simulink subsystem "AeroPropRefFranc"  (R2024b)
settings: Solver=VariableStepAuto  StartTime=0.0  StopTime=10.0  RelTol=1e-3
undefined symbols (not defined in the file or in its folder): ess, Force_b, Fprop_r, geom, H_b, Hdot_b, Moment_b, mot, mot2, mot3, mot4, Mprop_r, propel, propel2, propel3, propel4, pxf_diagram_options, SimIn, SimPar, tc, tc2, tc3, tc4
libraries: simulink x8, slpidlib x4, starslibAxisTransformations x2, libAxisTransformations x2
(part 1 of 10)
settings Model: Creator=drhill  LastModifiedBy=adcl
settings SolverCC: AlgebraicLoopSolver=TrustRegion
settings OptimizationCC: ReuseModelBlockBuffer=off
settings DebuggingCC: UnconnectedInputMsg=warning  UnconnectedOutputMsg=warning  UnconnectedLineMsg=warning
settings ModelReferenceCC: EnableRefExpFcnMdlSchedulingChecks=on
settings RTWCC: GPUComputeCapability=3.5  DLArmComputeVersion=19.05

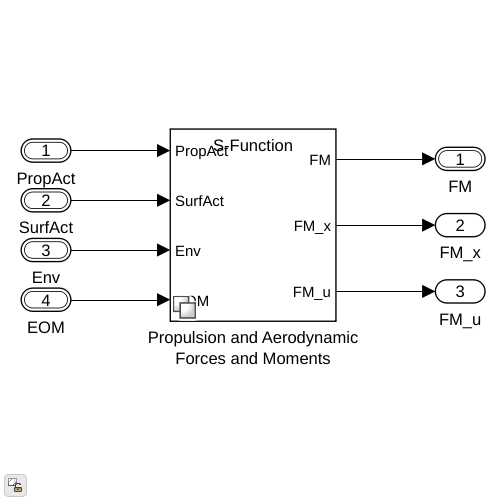
[thumbnail: Simulink's stored preview of the top-level diagram]
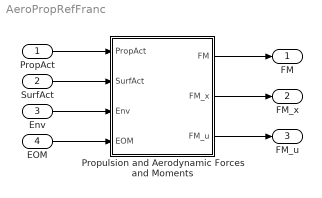
== system AeroPropRefFranc ==
  PropAct : Inport  OutDataTypeStr=Bus: BUS_PROP_ACTUATOR
  SurfAct : Inport  Port=2  OutDataTypeStr=Bus: BUS_SURF_ACTUATOR
  Env : Inport  Port=3  OutDataTypeStr=Bus: EnvironmentBus
  EOM : Inport  Port=4  OutDataTypeStr=Bus: EomBus
  Propulsion and Aerodynamic Forces and Moments : Subsystem  Variant=on  VariantControl=Variant1
  FM : Outport  OutDataTypeStr=Bus: ForceMomentBus
  FM_x : Outport  Port=2
  FM_u : Outport  Port=3
  wires:
  Propulsion and Aerodynamic Forces and Moments/1(FM) -> FM/1
  Env/1 -> Propulsion and Aerodynamic Forces and Moments/3(Env)
  SurfAct/1 -> Propulsion and Aerodynamic Forces and Moments/2(SurfAct)
  PropAct/1 -> Propulsion and Aerodynamic Forces and Moments/1(PropAct)
  EOM/1 -> Propulsion and Aerodynamic Forces and Moments/4(EOM)
  Propulsion and Aerodynamic Forces and Moments/2(FM_x) -> FM_x/1
  Propulsion and Aerodynamic Forces and Moments/3(FM_u) -> FM_u/1

== system AeroPropRefFranc/Propulsion and Aerodynamic Forces and Moments ==
  PropAct : Inport  OutDataTypeStr=Bus: BUS_PROP_ACTUATOR
  SurfAct : Inport  Port=2  OutDataTypeStr=Bus: BUS_SURF_ACTUATOR
  Env : Inport  Port=3  OutDataTypeStr=Bus: EnvironmentBus
  EOM : Inport  Port=4  OutDataTypeStr=Bus: EomBus
  Polynomial : Subsystem  VariantControl=GVS_FM_TYPE_POLYNOMIAL
  S-Function : Subsystem  VariantControl=GVS_FM_TYPE_SFUNCTION
  FM : Outport  OutDataTypeStr=Bus: ForceMomentBus
  FM_x : Outport  Port=2
  FM_u : Outport  Port=3

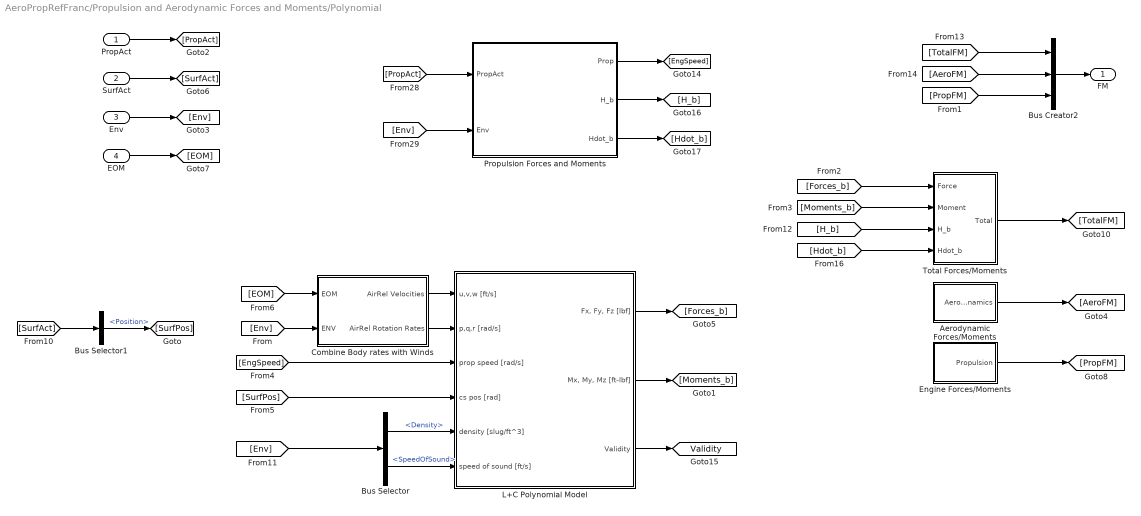
== system AeroPropRefFranc/Propulsion and Aerodynamic Forces and Moments/Polynomial ==
  PropAct : Inport  OutDataTypeStr=Bus: BUS_PROP_ACTUATOR
  SurfAct : Inport  Port=2  OutDataTypeStr=Bus: BUS_SURF_ACTUATOR
  Env : Inport  Port=3  OutDataTypeStr=Bus: EnvironmentBus
  EOM : Inport  Port=4  OutDataTypeStr=Bus: EomBus
  Aerodynamic Forces/Moments : Subsystem
  Bus Creator2 : BusCreator  Inputs=3  OutDataTypeStr=Bus: ForceMomentBus
  Bus Selector : BusSelector  OutputSignals=Atmosphere.Density,Atmosphere.SpeedOfSound
  Bus Selector1 : BusSelector  OutputSignals=Position
  Combine Body rates with Winds : Subsystem
  Engine Forces/Moments : Subsystem
  L+C Polynomial Model : Subsystem  VariantControl=AeroModel == gncAeroModel.GGA  mask{Model=SimIn.Model, Units=SimIn.Units}
      mask prompts: Model "Model Parameters"; Units "Unit Conversions"
  Propulsion Forces and Moments : Subsystem  VariantControl=GVS_PROP_TYPE_NONE
  Total Forces/Moments : Subsystem
  FM : Outport  OutDataTypeStr=Bus: ForceMomentBus  VectorParamsAs1DForOutWhenUnconnected=off
  tag scope: Validity=global
  wires:
  L+C Polynomial Model/3(Validity) -> [Validity]
  Bus Selector/1 -> L+C Polynomial Model/5(density [slug/ft^3])  "<Density>"
  [Env] -> Bus Selector/1
  [EngSpeed] -> L+C Polynomial Model/3(prop speed [rad/s])
  L+C Polynomial Model/1("Fx, Fy, Fz [lbf]") -> [Forces_b]
  [SurfPos] -> L+C Polynomial Model/4(cs pos [rad])
  L+C Polynomial Model/2("Mx, My, Mz [ft-lbf]") -> [Moments_b]
  Propulsion Forces and Moments/1(Prop) -> [EngSpeed]
  [H_b] -> Total Forces/Moments/3(H_b)
  [Env] -> Propulsion Forces and Moments/2(Env)
  [PropAct] -> Propulsion Forces and Moments/1(PropAct)
  [PropFM] -> Bus Creator2/3
  [AeroFM] -> Bus Creator2/2
  [TotalFM] -> Bus Creator2/1
  Propulsion Forces and Moments/2(H_b) -> [H_b]
  Propulsion Forces and Moments/3(Hdot_b) -> [Hdot_b]
  PropAct/1 -> [PropAct]
  Env/1 -> [Env]
  EOM/1 -> [EOM]
  SurfAct/1 -> [SurfAct]
  [SurfAct] -> Bus Selector1/1
  Bus Selector1/1 -> [SurfPos]  "<Position>"
  Bus Creator2/1 -> FM/1
  Aerodynamic Forces/Moments/1(Aerodynamics) -> [AeroFM]
  Engine Forces/Moments/1(Propulsion) -> [PropFM]
  Bus Selector/2 -> L+C Polynomial Model/6(speed of sound [ft/s])  "<SpeedOfSound>"
  Combine Body rates with Winds/1(AirRel Velocities) -> L+C Polynomial Model/1(u,v,w [ft/s])
  [EOM] -> Combine Body rates with Winds/1(EOM)
  [Env] -> Combine Body rates with Winds/2(ENV)
  [Forces_b] -> Total Forces/Moments/1(Force)
  [Moments_b] -> Total Forces/Moments/2(Moment)
  [Hdot_b] -> Total Forces/Moments/4(Hdot_b)
  Total Forces/Moments/1(Total) -> [TotalFM]
  Combine Body rates with Winds/2(AirRel Rotation Rates) -> L+C Polynomial Model/2(p,q,r [rad/s])

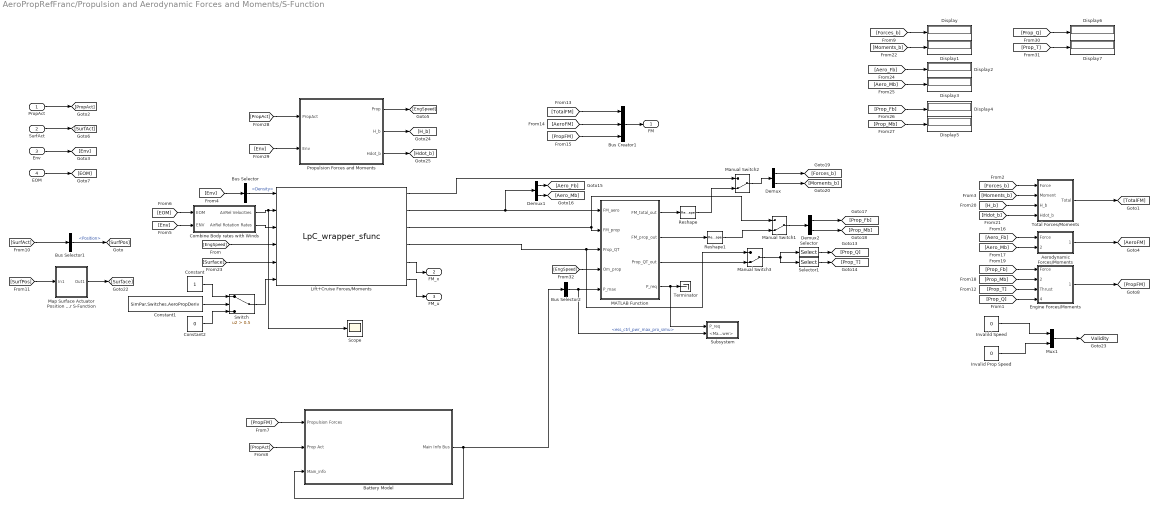
== system AeroPropRefFranc/Propulsion and Aerodynamic Forces and Moments/S-Function ==
  PropAct : Inport  OutDataTypeStr=Bus: BUS_PROP_ACTUATOR
  SurfAct : Inport  Port=2  OutDataTypeStr=Bus: BUS_SURF_ACTUATOR
  Env : Inport  Port=3  OutDataTypeStr=Bus: EnvironmentBus
  EOM : Inport  Port=4  OutDataTypeStr=Bus: EomBus
  Aerodynamic Forces/Moments : Subsystem
  Battery Model : Subsystem
  Bus Creator1 : BusCreator  Inputs=3  OutDataTypeStr=Bus: ForceMomentBus
  Bus Selector : BusSelector  OutputSignals=Atmosphere.Density
  Bus Selector1 : BusSelector  OutputSignals=Position
  Bus Selector2 : BusSelector  OutputSignals=ctrl.ess_ctrl_pwr_max_pro_simu
  Combine Body rates with Winds : Subsystem
  Constant : Constant
  Constant1 : Constant  Value=SimPar.Switches.AeroPropDeriv
  Constant2 : Constant  Value=0
  Demux : Demux  Outputs=[3 3]
  Demux1 : Demux  Outputs=[3 3]
  Demux2 : Demux  Outputs=[3 3]
  Display{,1..7} (8 alike) : Display
  Engine Forces/Moments : Subsystem
  Invalid Prop Speed : Constant  Value=0
  Invalild Speed : Constant  Value=0
  Lift+Cruise Forces/Moments : S-Function  FunctionName=LpC_wrapper_sfunc  SFunctionDeploymentMode=off  EnableBusSupport=off
      mask Display:
      | port_label('input',1,'air density');
      | port_label('input',2,'Velocity, body');
      | port_label('input',3,'Angular Rates, body');
      | port_label('input',4,'Engine Speeds');
      | port_label('input',5,'Surface Deflections');
      | port_label('input',6,'Compute Derivatives');
      | port_label('output',1,'Total Forces/Moments');
      | port_label('output',2,'Aero Total Forces/Moments');
      | port_label('output',3,'Prop Forces/Moments');
      | port_label('output',4,'Prop Torque/Thrust');
      | port_label('output',5,'FM_x');
      | port_label('output',6,'FM_u');
  MATLAB Function : MATLAB Function  TreatAsAtomicUnit=on
  Manual Switch1 : ManualSwitch  CurrentSetting=0
  Manual Switch2 : ManualSwitch  CurrentSetting=0
  Manual Switch3 : ManualSwitch  CurrentSetting=0
  Map Surface Actuator Position To Surface Inputs for S-Function : Subsystem
  Mux1 : Mux  Inputs=2
  Propulsion Forces and Moments : Subsystem  VariantControl=GVS_PROP_TYPE_NONE
  Reshape : Reshape
  Reshape1 : Reshape
  Scope : Scope
  Selector : Selector  NumberOfDimensions=2  InputPortWidth=3  IndexOptions=Index vector (dialog),Select all  Indices=1,1  OutputSizes=1,1
  Selector1 : Selector  NumberOfDimensions=2  InputPortWidth=3  IndexOptions=Index vector (dialog),Select all  Indices=2,1  OutputSizes=1,1
  Subsystem : Subsystem
  Switch : Switch  Criteria=u2 > Threshold  Threshold=0.5  OutDataTypeStr=boolean  SaturateOnIntegerOverflow=off  InputSameDT=off
  Terminator : Terminator
  Total Forces/Moments : Subsystem
  FM : Outport  OutDataTypeStr=Bus: ForceMomentBus  VectorParamsAs1DForOutWhenUnconnected=off
  FM_x : Outport  Port=2
  FM_u : Outport  Port=3
  tag scope: Validity=global
  wires:
  MATLAB Function/4(P_req) -> Terminator/1, Subsystem/1(P_req)
  Bus Selector2/1 -> MATLAB Function/5(P_max), Subsystem/2(<Max Power>)  "<ess_ctrl_pwr_max_pro_simu>"
  [EngSpeed] -> MATLAB Function/4(Om_prop)
  MATLAB Function/3(Prop_QT_out) -> Manual Switch3/2
  Lift+Cruise Forces/Moments/4 -> Manual Switch3/1, MATLAB Function/3(Prop_QT)
  Manual Switch3/1 -> Selector/1, Selector1/1
  Manual Switch1/1 -> Demux2/1
  Reshape/1 -> Manual Switch2/2
  Manual Switch2/1 -> Demux/1
  Reshape1/1 -> Manual Switch1/2
  MATLAB Function/2(FM_prop_out) -> Reshape1/1
  Lift+Cruise Forces/Moments/2 -> Demux1/1, MATLAB Function/1(FM_aero)
  MATLAB Function/1(FM_total_out) -> Reshape/1
  Battery Model/1(Main Info Bus) -> Bus Selector2/1, Battery Model/3(Main_info)
  [PropAct] -> Battery Model/2(Prop Act)
  [PropFM] -> Battery Model/1(Propulsion Forces)
  Lift+Cruise Forces/Moments/6 -> FM_u/1
  Lift+Cruise Forces/Moments/5 -> FM_x/1
  PropAct/1 -> [PropAct]
  Env/1 -> [Env]
  EOM/1 -> [EOM]
  SurfAct/1 -> [SurfAct]
  [EngSpeed] -> Lift+Cruise Forces/Moments/4
  Constant2/1 -> Switch/3
  [Surface] -> Lift+Cruise Forces/Moments/5
  Constant/1 -> Switch/1
  [Env] -> Bus Selector/1
  Bus Selector/1 -> Lift+Cruise Forces/Moments/1  "<Density>"
  Propulsion Forces and Moments/3(Hdot_b) -> [Hdot_b]
  [EOM] -> Combine Body rates with Winds/1(EOM)
  Propulsion Forces and Moments/2(H_b) -> [H_b]
  Propulsion Forces and Moments/1(Prop) -> [EngSpeed]
  [PropAct] -> Propulsion Forces and Moments/1(PropAct)
  [Env] -> Propulsion Forces and Moments/2(Env)
  [SurfAct] -> Bus Selector1/1
  Bus Selector1/1 -> [SurfPos]  "<Position>"
  Bus Creator1/1 -> FM/1
  [TotalFM] -> Bus Creator1/1
  [AeroFM] -> Bus Creator1/2
  [PropFM] -> Bus Creator1/3
  Total Forces/Moments/1(Total) -> [TotalFM]
  Aerodynamic Forces/Moments/1(Aerodynamics) -> [AeroFM]
  Engine Forces/Moments/1(Propulsion) -> [PropFM]
  [Moments_b] -> Total Forces/Moments/2(Moment)
  [Forces_b] -> Total Forces/Moments/1(Force)
  [SurfPos] -> Map Surface Actuator Position To Surface Inputs for S-Function/1(In1)
  Map Surface Actuator Position To Surface Inputs for S-Function/1(Out1) -> [Surface]
  [Prop_Q] -> Engine Forces/Moments/4(Torque)
  [Prop_T] -> Engine Forces/Moments/3(Thrust)
  Lift+Cruise Forces/Moments/1 -> Manual Switch2/1
  Lift+Cruise Forces/Moments/3 -> Manual Switch1/1, MATLAB Function/2(FM_prop)
  Demux/1 -> [Forces_b]
  Demux/2 -> [Moments_b]
  Selector1/1 -> [Prop_T]
  Selector/1 -> [Prop_Q]
  Demux1/1 -> [Aero_Fb]
  Demux1/2 -> [Aero_Mb]
  Demux2/1 -> [Prop_Fb]
  Demux2/2 -> [Prop_Mb]
  [Prop_Fb] -> Engine Forces/Moments/1(Force)
  [Prop_Mb] -> Engine Forces/Moments/2(Moment)
  [Aero_Fb] -> Aerodynamic Forces/Moments/1(Force)
  [Aero_Mb] -> Aerodynamic Forces/Moments/2(Moment)
  Mux1/1 -> [Validity]
  Invalild Speed/1 -> Mux1/1
  Invalid Prop Speed/1 -> Mux1/2
  Constant1/1 -> Switch/2
  [Env] -> Combine Body rates with Winds/2(ENV)
  Combine Body rates with Winds/1(AirRel Velocities) -> Lift+Cruise Forces/Moments/2, Scope/1
  Combine Body rates with Winds/2(AirRel Rotation Rates) -> Lift+Cruise Forces/Moments/3
  Switch/1 -> Lift+Cruise Forces/Moments/6
  [H_b] -> Total Forces/Moments/3(H_b)
  [Hdot_b] -> Total Forces/Moments/4(Hdot_b)
  [Forces_b] -> Display/1
  [Moments_b] -> Display1/1
  [Aero_Fb] -> Display2/1
  [Aero_Mb] -> Display3/1
  [Prop_Fb] -> Display4/1
  [Prop_Mb] -> Display5/1
  [Prop_Q] -> Display6/1
  [Prop_T] -> Display7/1

== system AeroPropRefFranc/Propulsion and Aerodynamic Forces and Moments/Polynomial/Aerodynamic Forces//Moments ==
  RenameAeroForceMomentBus : Subsystem
  Aerodynamics : Outport
  wires:
  RenameAeroForceMomentBus/1(Aerodynamics) -> Aerodynamics/1

== system AeroPropRefFranc/Propulsion and Aerodynamic Forces and Moments/Polynomial/Combine Body rates with Winds ==
  note: Combine Vehicle Inertial velocities/ rotational rates with winds and turbulence
  EOM : Inport
  ENV : Inport  Port=2
  Add : Sum  Inputs=+++
  Add1 : Sum
  Bus Selector3 : BusSelector  OutputSignals=Wind.Vel_wHh,Turbulence.Vel_tBb,Turbulence.Omeg_TBb
  Bus Selector4 : BusSelector  OutputSignals=InertialData.Vel_bIi,InertialData.Omeg_BIb,InertialData.Q_i2b,WorldRelativeData.Q_h2b
  Quaternion Vector Transformation : starslibAxisTransformations/Quaternion Vector Transformation  n=0
  Quaternion Vector Transformation1 : starslibAxisTransformations/Quaternion Vector Transformation  n=0
  AirRel Velocities : Outport
  AirRel Rotation Rates : Outport  Port=2
  wires:
  [Q_h2b] -> Quaternion Vector Transformation1/1  "Moment_b"
  [Omeg_BIb] -> Add1/2  "Force_b"
  Add1/1 -> AirRel Rotation Rates/1  "Total"
  Add/1 -> AirRel Velocities/1
  Bus Selector3/3 -> Add1/1  "<Omeg_TBb>"
  Bus Selector3/2 -> [Vel_turb_body]  "<Vel_tBb>"
  Bus Selector4/2 -> [Omeg_BIb]  "<Omeg_BIb>"
  Bus Selector4/3 -> [Q_i2b]  "<Q_i2b>"
  Bus Selector4/4 -> [Q_h2b]  "<Q_h2b>"
  Bus Selector4/1 -> [Vel_bIi]  "<Vel_bIi>"
  ENV/1 -> Bus Selector3/1
  EOM/1 -> Bus Selector4/1
  [Vel_wind_body] -> Add/2
  [Vel_bIi] -> Quaternion Vector Transformation/2
  [Vel_bIb] -> Add/1
  [Vel_turb_body] -> Add/3
  [Q_i2b] -> Quaternion Vector Transformation/1
  Bus Selector3/1 -> Quaternion Vector Transformation1/2  "<Vel_wHh>"
  Quaternion Vector Transformation1/1 -> [Vel_wind_body]
  Quaternion Vector Transformation/1 -> [Vel_bIb]

== system AeroPropRefFranc/Propulsion and Aerodynamic Forces and Moments/Polynomial/Engine Forces//Moments ==
  RenameEngineForceMomentBus : Subsystem
  Propulsion : Outport
  wires:
  RenameEngineForceMomentBus/1(Propulsion) -> Propulsion/1

== system AeroPropRefFranc/Propulsion and Aerodynamic Forces and Moments/Polynomial/L+C Polynomial Model ==
  note: Control surface positions
      | 1-2: L,R Aileron
      | 3-4: L,R Elevator
      | 5: Rudder
  note: controls
  note: states
  note: atmosphere
  u,v,w [ft/s] : Inport
  p,q,r [rad/s] : Inport  Port=2
  prop speed [rad/s] : Inport  Port=3
  cs pos [rad] : Inport  Port=4
  density [slug/ft^3] : Inport  Port=5
  speed of sound [ft/s] : Inport  Port=6
  Data Type Conversion : DataTypeConversion  SaturateOnIntegerOverflow=off  RndMeth=Floor
  L+C Aerodynamic Model : MATLAB Function  TreatAsAtomicUnit=on
  Mux : Mux  Inputs=2
  "Fx, Fy, Fz [lbf]" : Outport
  "Mx, My, Mz [ft-lbf]" : Outport  Port=2
  Validity : Outport  Port=3  OutDataTypeStr=double  PortDimensions=[1 2]
  wires:
  Data Type Conversion/1 -> Validity/1
  speed of sound [ft/s]/1 -> L+C Aerodynamic Model/5(a)
  L+C Aerodynamic Model/3(Validity) -> Data Type Conversion/1
  Mux/1 -> L+C Aerodynamic Model/1(x)
  cs pos [rad]/1 -> L+C Aerodynamic Model/3(d)
  prop speed [rad/s]/1 -> L+C Aerodynamic Model/2(n)
  p,q,r [rad/s]/1 -> Mux/2
  u,v,w [ft/s]/1 -> Mux/1
  L+C Aerodynamic Model/1(Fb) -> "Fx, Fy, Fz [lbf]"/1
  L+C Aerodynamic Model/2(Mb) -> "Mx, My, Mz [ft-lbf]"/1
  density [slug/ft^3]/1 -> L+C Aerodynamic Model/4(rho)

== system AeroPropRefFranc/Propulsion and Aerodynamic Forces and Moments/Polynomial/Propulsion Forces and Moments ==
  PropAct : Inport
  Env : Inport  Port=2
  Bus Selector : BusSelector  OutputSignals=EngSpeed,EngAccel
  Bus Selector5 : BusSelector  OutputSignals=Atmosphere
  Reshape : Reshape  OutputDimensionality=Column vector (2-D)
  Reshape1 : Reshape  OutputDimensionality=Column vector (2-D)
  Terminator2 : Terminator
  Total Angular Momentum : Subsystem  mask{Model=SimIn.Model}
      mask prompts: Model "Modeling Parameters"
  Prop : Outport  VectorParamsAs1DForOutWhenUnconnected=off
  H_b : Outport  Port=2  VectorParamsAs1DForOutWhenUnconnected=off
  Hdot_b : Outport  Port=3  VectorParamsAs1DForOutWhenUnconnected=off
  wires:
  Reshape1/1 -> [Hdot_b]  "Hdot_b"
  Reshape/1 -> [H_b]  "H_b"
  [Atmos] -> Terminator2/1
  [EngSpeed] -> Prop/1
  Env/1 -> [Env]
  PropAct/1 -> [PropAct]
  Bus Selector5/1 -> [Atmos]  "<Atmosphere>"
  Bus Selector/1 -> [EngSpeed]  "<EngSpeed>"
  Bus Selector/2 -> [EngAccel]  "<EngAccel>"
  [PropAct] -> Bus Selector/1
  [Env] -> Bus Selector5/1
  [EngAccel] -> Total Angular Momentum/2(EngAccel)
  [EngSpeed] -> Total Angular Momentum/1(EngSpeed)
  Total Angular Momentum/1(H_b) -> Reshape/1
  Total Angular Momentum/2(Hdot_b) -> Reshape1/1
  [H_b] -> H_b/1
  [Hdot_b] -> Hdot_b/1

== system AeroPropRefFranc/Propulsion and Aerodynamic Forces and Moments/Polynomial/Total Forces//Moments ==
  Force : Inport
  Moment : Inport  Port=2
  H_b : Inport  Port=3
  Hdot_b : Inport  Port=4
  Bus Assignment : BusAssignment  AssignedSignals=Force_b,Moment_b,H_b,Hdot_b
  RenameTotalForceMomentBus : Subsystem
  Reshape : Reshape
  Reshape1 : Reshape
  Total : Outport
  wires:
  Reshape1/1 -> Bus Assignment/5
  Reshape/1 -> Bus Assignment/4
  [H_b] -> Reshape/1  "H_b"
  [Hdot_b] -> Reshape1/1  "Hdot_b"
  H_b/1 -> [H_b]
  Hdot_b/1 -> [Hdot_b]
  [Moments_b] -> Bus Assignment/3  "Moment_b"
  RenameTotalForceMomentBus/1(Total) -> Bus Assignment/1
  [Forces_b] -> Bus Assignment/2  "Force_b"
  Bus Assignment/1 -> Total/1  "Total"
  Moment/1 -> [Moments_b]
  Force/1 -> [Forces_b]

== system AeroPropRefFranc/Propulsion and Aerodynamic Forces and Moments/S-Function/Aerodynamic Forces//Moments ==
  Force : Inport
  Moment : Inport  Port=2
  Bus Assignment : BusAssignment  AssignedSignals=Force_b,Moment_b
  RenameAeroForceMomentBus : Subsystem
  Aerodynamics : Outport
  wires:
  Force/1 -> [Aero_Fb]
  Moment/1 -> [Aero_Mb]
  RenameAeroForceMomentBus/1(Aerodynamics) -> Bus Assignment/1
  [Aero_Fb] -> Bus Assignment/2
  [Aero_Mb] -> Bus Assignment/3
  Bus Assignment/1 -> Aerodynamics/1  "Aerodynamics"

== system AeroPropRefFranc/Propulsion and Aerodynamic Forces and Moments/S-Function/Battery Model ==
  Propulsion Forces : Inport
  Prop Act : Inport  Port=2
  Main_info : Inport  Port=3
  Bus Selector : BusSelector  OutputSignals=Mprop_r
  Bus Selector1 : BusSelector  OutputSignals=EngSpeed
  Bus Selector2 : BusSelector  OutputSignals=plant.ess_plant_curr_out_simu,plant.ess_plant_volt_out_simu
  Demux : Demux  Outputs=9
  Display : Display
  Gain : Gain  Gain=-1
  Ground : Ground
  Ground_7 : Ground
  Product : Product
  Product1 : Product
  Reciprocal : Product  Inputs=/
  Subsystem : Subsystem
  Subsystem1 : Subsystem
  Subsystem2 : Subsystem
  Sum : Sum  Inputs=++++++++++
  Terminator{,1..4} (5 alike) : Terminator
  accelec : Subsystem
  ess (battery) : Subsystem
  powerplant : Subsystem  Commented=on
  Main Info Bus : Outport
  wires:
  Main_info/1 -> ess (battery)/1(main_info_bus_in)
  accelec/2(system_effort_out) -> Terminator4/1
  accelec/1(system_bus_out) -> Terminator3/1  "accelec"
  accelec/3(system_flow_out) -> Display/1, Sum/10
  Ground/1 -> accelec/3(system_flow_in)
  ess (battery)/2(system_effort_out) -> accelec/2(system_effort_in)
  Bus Selector2/1 -> Terminator2/1  "<ess_plant_curr_out_simu>"
  Subsystem1/1(Out1) -> Terminator/1
  Subsystem/1(Current) -> Terminator1/1
  Gain/1 -> Product/1
  Reciprocal/1 -> Product1/2
  Bus Selector2/2 -> Reciprocal/1  "<ess_plant_volt_out_simu>"
  Product1/1 -> Demux/1, Subsystem/1(Current_each)  "Current"
  ess (battery)/1(system_bus_out) -> Main Info Bus/1, accelec/1(main_info_bus_in), Bus Selector2/1, Subsystem2/1(system_bus_out)  "ess"
  Sum/1 -> ess (battery)/3(system_flow_in), Subsystem/2(Current_total)  "Current_total"
  Demux/9 -> Sum/9  "Current9"
  Demux/8 -> Sum/8  "Current8"
  Demux/7 -> Sum/7  "Current7"
  Demux/6 -> Sum/6  "Current6"
  Demux/5 -> Sum/5  "Current5"
  Demux/4 -> Sum/4  "Current4"
  Demux/3 -> Sum/3  "Current3"
  Demux/2 -> Sum/2  "Current2"
  Demux/1 -> Sum/1  "Current1"
  Product/1 -> Subsystem1/1(In1), Product1/1
  Bus Selector/1 -> Gain/1  "<Mprop_r>"
  Bus Selector1/1 -> Product/2  "<EngSpeed>"
  Prop Act/1 -> Bus Selector1/1
  Propulsion Forces/1 -> Bus Selector/1
  Ground_7/1 -> ess (battery)/2(system_effort_in)

== system AeroPropRefFranc/Propulsion and Aerodynamic Forces and Moments/S-Function/Combine Body rates with Winds ==
  note: Combine Vehicle Inertial velocities/ rotational rates with winds and turbulence
  EOM : Inport
  ENV : Inport  Port=2
  Add : Sum  Inputs=+++
  Add1 : Sum
  Bus Selector3 : BusSelector  OutputSignals=Wind.Vel_wHh,Turbulence.Vel_tBb,Turbulence.Omeg_TBb
  Bus Selector4 : BusSelector  OutputSignals=InertialData.Vel_bIi,InertialData.Omeg_BIb,InertialData.Q_i2b,WorldRelativeData.Q_h2b
  Quaternion Vector Transformation : libAxisTransformations/Quaternion Vector Transformation  n=0
  Quaternion Vector Transformation1 : libAxisTransformations/Quaternion Vector Transformation  n=0
  Scope : Scope
  AirRel Velocities : Outport
  AirRel Rotation Rates : Outport  Port=2
  wires:
  [Vel_wind_body] -> Add/2
  [Vel_turb_body] -> Add/3, Scope/1
  EOM/1 -> Bus Selector4/1
  Quaternion Vector Transformation1/1 -> [Vel_wind_body]
  ENV/1 -> Bus Selector3/1
  Bus Selector3/2 -> [Vel_turb_body]  "<Vel_tBb>"
  [Q_i2b] -> Quaternion Vector Transformation/1
  Bus Selector3/3 -> Add1/1  "<Omeg_TBb>"
  Quaternion Vector Transformation/1 -> [Vel_bIb]
  Bus Selector3/1 -> Quaternion Vector Transformation1/2  "<Vel_wHh>"
  Bus Selector4/4 -> [Q_h2b]  "<Q_h2b>"
  [Q_h2b] -> Quaternion Vector Transformation1/1
  [Vel_bIi] -> Quaternion Vector Transformation/2
  [Vel_bIb] -> Add/1
  [Omeg_BIb] -> Add1/2
  Bus Selector4/3 -> [Q_i2b]  "<Q_i2b>"
  Add1/1 -> AirRel Rotation Rates/1
  Bus Selector4/1 -> [Vel_bIi]  "<Vel_bIi>"
  Bus Selector4/2 -> [Omeg_BIb]  "<Omeg_BIb>"
  Add/1 -> AirRel Velocities/1

== system AeroPropRefFranc/Propulsion and Aerodynamic Forces and Moments/S-Function/Engine Forces//Moments ==
  Force : Inport
  Moment : Inport  Port=2
  Thrust : Inport  Port=3
  Torque : Inport  Port=4
  Bus Assignment : BusAssignment  AssignedSignals=Force_b,Moment_b,Fprop_r,Mprop_r
  RenameEngineForceMomentBus : Subsystem
  Reshape : Reshape
  Reshape1 : Reshape
  Propulsion : Outport
  wires:
  Moment/1 -> [Prop_Mb]
  RenameEngineForceMomentBus/1(Propulsion) -> Bus Assignment/1
  Bus Assignment/1 -> Propulsion/1  "Propulsion"
  [Prop_Fb] -> Bus Assignment/2
  Force/1 -> [Prop_Fb]
  [Prop_Mb] -> Bus Assignment/3
  Thrust/1 -> [Prop_T]
  Torque/1 -> [Prop_Q]
  [Prop_T] -> Reshape/1
  [Prop_Q] -> Reshape1/1
  Reshape/1 -> Bus Assignment/4
  Reshape1/1 -> Bus Assignment/5

== system AeroPropRefFranc/Propulsion and Aerodynamic Forces and Moments/S-Function/Map Surface Actuator Position To Surface Inputs for S-Function ==
  note: Note:  Assumes left and right aileron position are the same,
      |           which would not be the case if one failed
  In1 : Inport
  Demux : Demux  Outputs=SimIn.numSurfaces
  Gain : Gain  Gain=0.5
  Gain1 : Gain  Gain=0.5
  Gain2 : Gain  Gain=0.5
  Mux1 : Mux
  Sum : Sum
  Sum1 : Sum
  Sum2 : Sum  Inputs=+-
  Out1 : Outport
  wires:
  [RFA] -> Sum2/1
  [LFA] -> Sum2/2
  Sum2/1 -> Gain2/1
  Gain2/1 -> [Aileron]  "Aileron"
  Gain1/1 -> [Flap]  "Flap"
  [Elevator] -> Mux1/3
  [LE] -> Sum/1
  [Flap] -> Mux1/2
  Demux/1 -> [LFA]  "Left Flaperon"
  Mux1/1 -> Out1/1
  [RFA] -> Sum1/2
  Demux/2 -> [RFA]  "Right Flaperon"
  Demux/5 -> [Rudder]  "Rudder"
  [Aileron] -> Mux1/1
  [Rudder] -> Mux1/4
  Gain/1 -> [Elevator]  "Elevator"
  Demux/4 -> [RE]  "Right Elevator"
  Sum1/1 -> Gain1/1
  [LFA] -> Sum1/1
  Demux/3 -> [LE]  "Left Elevator"
  [RE] -> Sum/2
  Sum/1 -> Gain/1
  In1/1 -> Demux/1

== system AeroPropRefFranc/Propulsion and Aerodynamic Forces and Moments/S-Function/Propulsion Forces and Moments ==
  PropAct : Inport
  Env : Inport  Port=2
  Bus Selector : BusSelector  OutputSignals=EngSpeed,EngAccel
  Bus Selector5 : BusSelector  OutputSignals=Atmosphere
  Terminator2 : Terminator
  Total Angular Momentum : Subsystem  mask{Model=SimIn.CModel}
      mask prompts: Model "Modeling Parameters"
  Prop : Outport  VectorParamsAs1DForOutWhenUnconnected=off
  H_b : Outport  Port=2  VectorParamsAs1DForOutWhenUnconnected=off
  Hdot_b : Outport  Port=3  VectorParamsAs1DForOutWhenUnconnected=off
  wires:
  PropAct/1 -> [PropAct]
  Env/1 -> [Env]
  [EngSpeed] -> Prop/1
  [Atmos] -> Terminator2/1
  Bus Selector5/1 -> [Atmos]  "<Atmosphere>"
  Bus Selector/1 -> [EngSpeed]  "<EngSpeed>"
  Bus Selector/2 -> [EngAccel]  "<EngAccel>"
  [PropAct] -> Bus Selector/1
  [Env] -> Bus Selector5/1
  [EngAccel] -> Total Angular Momentum/2(EngAccel)
  [EngSpeed] -> Total Angular Momentum/1(EngSpeed)
  Total Angular Momentum/1(H_b) -> [H_b]
  Total Angular Momentum/2(Hdot_b) -> [Hdot_b]
  [H_b] -> H_b/1
  [Hdot_b] -> Hdot_b/1

== system AeroPropRefFranc/Propulsion and Aerodynamic Forces and Moments/S-Function/Subsystem ==
  P_req : Inport
  <Max Power> : Inport  Port=2
  Bus Creator : BusCreator  Inputs=2
  Terminator : Terminator
  wires:
  Bus Creator/1 -> Terminator/1  "Motor_Power"
  <Max Power>/1 -> Bus Creator/2  "Max_Power"
  P_req/1 -> Bus Creator/1  "Current_Power"

== system AeroPropRefFranc/Propulsion and Aerodynamic Forces and Moments/S-Function/Total Forces//Moments ==
  Force : Inport
  Moment : Inport  Port=2
  H_b : Inport  Port=3
  Hdot_b : Inport  Port=4
  Bus Assignment : BusAssignment  AssignedSignals=Force_b,Moment_b,H_b,Hdot_b
  RenameTotalForceMomentBus : Subsystem
  Total : Outport
  wires:
  RenameTotalForceMomentBus/1(Total) -> Bus Assignment/1
  Bus Assignment/1 -> Total/1  "Total"
  Moment/1 -> [Moments_b]
  Force/1 -> [Forces_b]
  [Forces_b] -> Bus Assignment/2
  [Moments_b] -> Bus Assignment/3
  [Hdot_b] -> Bus Assignment/5
  [H_b] -> Bus Assignment/4
  H_b/1 -> [H_b]
  Hdot_b/1 -> [Hdot_b]

== system AeroPropRefFranc/Propulsion and Aerodynamic Forces and Moments/Polynomial/Aerodynamic Forces//Moments/RenameAeroForceMomentBus ==
  Bus Creator2 : BusCreator  Inputs=2  OutDataTypeStr=Bus: AeroFMBus
  Constant2 : Constant  Value=zeros(3,1)
  Constant3 : Constant  Value=zeros(3,1)
  Aerodynamics : Outport
  wires:
  Constant3/1 -> Bus Creator2/2  "Moment_b"
  Constant2/1 -> Bus Creator2/1  "Force_b"
  Bus Creator2/1 -> Aerodynamics/1  "Aerodynamics"

== system AeroPropRefFranc/Propulsion and Aerodynamic Forces and Moments/Polynomial/Engine Forces//Moments/RenameEngineForceMomentBus ==
  Bus Creator2 : BusCreator  Inputs=11  OutDataTypeStr=Bus: EngineFMBus
  Constant{1..4} (4 alike) : Constant  Value=zeros(3,1)
  Constant{5..11} (7 alike) : Constant  Value=zeros(SimIn.numEngines,1)
  Propulsion : Outport
  wires:
  Constant3/1 -> Bus Creator2/2  "Moment_b"
  Constant2/1 -> Bus Creator2/1  "Force_b"
  Bus Creator2/1 -> Propulsion/1  "Propulsion"
  Constant1/1 -> Bus Creator2/3  "H_b"
  Constant4/1 -> Bus Creator2/4  "Hdot_b"
  Constant5/1 -> Bus Creator2/5  "Fprop_r"
  Constant6/1 -> Bus Creator2/6  "Mprop_r"
  Constant7/1 -> Bus Creator2/7  "Mmotor_r"
  Constant8/1 -> Bus Creator2/8  "Hdot_r"
  Constant9/1 -> Bus Creator2/9  "H_r"
  Constant10/1 -> Bus Creator2/10  "Omega_r"
  Constant11/1 -> Bus Creator2/11  "AdvanceRatio"

== system AeroPropRefFranc/Propulsion and Aerodynamic Forces and Moments/Polynomial/Propulsion Forces and Moments/Total Angular Momentum ==
  EngSpeed : Inport
  EngAccel : Inport  Port=2
  MATLAB Function : MATLAB Function  TreatAsAtomicUnit=on
  H_b : Outport
  Hdot_b : Outport  Port=2
  wires:
  MATLAB Function/2(Hdot_b) -> Hdot_b/1
  MATLAB Function/1(H_b) -> H_b/1
  EngAccel/1 -> MATLAB Function/2(EngAccel)
  EngSpeed/1 -> MATLAB Function/1(EngSpeed)

== system AeroPropRefFranc/Propulsion and Aerodynamic Forces and Moments/Polynomial/Total Forces//Moments/RenameTotalForceMomentBus ==
  Bus Creator2 : BusCreator  Inputs=4  OutDataTypeStr=Bus: TotalFMBus
  Constant{2..5} (4 alike) : Constant  Value=zeros(3,1)
  Total : Outport
  wires:
  Constant2/1 -> Bus Creator2/1  "Force_b"
  Constant3/1 -> Bus Creator2/2  "Moment_b"
  Constant5/1 -> Bus Creator2/4  "Hdot_b"
  Constant4/1 -> Bus Creator2/3  "H_b"
  Bus Creator2/1 -> Total/1  "Total"

== system AeroPropRefFranc/Propulsion and Aerodynamic Forces and Moments/S-Function/Aerodynamic Forces//Moments/RenameAeroForceMomentBus ==
  Bus Creator2 : BusCreator  Inputs=2  OutDataTypeStr=Bus: AeroFMBus
  Constant2 : Constant  Value=zeros(3,1)
  Constant3 : Constant  Value=zeros(3,1)
  Aerodynamics : Outport
  wires:
  Constant3/1 -> Bus Creator2/2  "Moment_b"
  Constant2/1 -> Bus Creator2/1  "Force_b"
  Bus Creator2/1 -> Aerodynamics/1  "Aerodynamics"

== system AeroPropRefFranc/Propulsion and Aerodynamic Forces and Moments/S-Function/Battery Model/Subsystem ==
  Current_each : Inport
  Current_total : Inport  Port=2
  Bus Creator : BusCreator  Inputs=10
  Demux : Demux  Outputs=9
  Current : Outport
  wires:
  Demux/9 -> Bus Creator/9  "Current9"
  Demux/8 -> Bus Creator/8  "Current8"
  Demux/7 -> Bus Creator/7  "Current7"
  Demux/6 -> Bus Creator/6  "Current6"
  Demux/5 -> Bus Creator/5  "Current5"
  Demux/4 -> Bus Creator/4  "Current4"
  Demux/3 -> Bus Creator/3  "Current3"
  Demux/2 -> Bus Creator/2  "Current2"
  Demux/1 -> Bus Creator/1  "Current1"
  Current_each/1 -> Demux/1
  Current_total/1 -> Bus Creator/10
  Bus Creator/1 -> Current/1  "Current"

== system AeroPropRefFranc/Propulsion and Aerodynamic Forces and Moments/S-Function/Battery Model/Subsystem1 ==
  In1 : Inport
  Bus Creator : BusCreator  Inputs=9
  Demux : Demux  Outputs=9
  Out1 : Outport
  wires:
  Bus Creator/1 -> Out1/1  "Power"
  Demux/9 -> Bus Creator/9  "Power9"
  Demux/8 -> Bus Creator/8  "Power8"
  Demux/7 -> Bus Creator/7  "Power7"
  Demux/6 -> Bus Creator/6  "Power6"
  Demux/5 -> Bus Creator/5  "Power5"
  Demux/4 -> Bus Creator/4  "Power4"
  Demux/3 -> Bus Creator/3  "Power3"
  Demux/2 -> Bus Creator/2  "Power2"
  Demux/1 -> Bus Creator/1  "Power1"
  In1/1 -> Demux/1

== system AeroPropRefFranc/Propulsion and Aerodynamic Forces and Moments/S-Function/Battery Model/Subsystem2 ==
  system_bus_out : Inport
  Bus Creator : BusCreator  Inputs=4
  Bus Selector : BusSelector  OutputSignals=plant.ess_plant_volt_out_simu,plant.ess_plant_curr_out_simu,plant.ess_plant_soc_simu
  Derivative : Derivative
  Gain : Gain
  Gain1 : Gain
  Gain2 : Gain  Gain=100
  Scope : Scope  Commented=on
  Terminator : Terminator
  To Workspace : ToWorkspace  VariableName=SOC  SaveFormat=Timeseries  SampleTime=-1
  To Workspace1 : ToWorkspace  VariableName=SOCRate  SaveFormat=Timeseries  SampleTime=-1
  wires:
  Derivative/1 -> Bus Creator/4, To Workspace1/1  "rate"
  Bus Creator/1 -> Terminator/1  "Battery_info"
  Gain2/1 -> Bus Creator/3, Derivative/1, To Workspace/1, Scope/1  "State of Charge"
  Bus Selector/3 -> Gain2/1  "<ess_plant_soc_simu>"
  Gain/1 -> Bus Creator/1  "Voltage"
  Gain1/1 -> Bus Creator/2  "Current"
  Bus Selector/2 -> Gain1/1  "<ess_plant_curr_out_simu>"
  Bus Selector/1 -> Gain/1  "<ess_plant_volt_out_simu>"
  system_bus_out/1 -> Bus Selector/1

== system AeroPropRefFranc/Propulsion and Aerodynamic Forces and Moments/S-Function/Battery Model/accelec ==
  main_info_bus_in : Inport
  system_effort_in : Inport  Port=2
  system_flow_in : Inport  Port=3
  Ground_1 : Ground
  Terminator_1 : Terminator
  plant : Subsystem
      mask Display: disp('accelec_plant_const_pwrloss_volt_in_nokey.slx')
  system_bus_out : Outport
  system_effort_out : Outport  Port=2
  system_flow_out : Outport  Port=3
  wires:
  plant/2(aOutport--2) -> Terminator_1/1
  Ground_1/1 -> plant/2(aInport--2)
  [plant] -> system_bus_out/1  "plant"
  system_flow_in/1 -> plant/4(in-flow-3)
  system_effort_in/1 -> plant/3(in-effort-2)
  plant/4(out-flow-7) -> system_flow_out/1
  plant/3(out-effort-6) -> system_effort_out/1
  plant/1(outport-system_info_bus) -> [plant]
  main_info_bus_in/1 -> plant/1(aInport--1)

== system AeroPropRefFranc/Propulsion and Aerodynamic Forces and Moments/S-Function/Battery Model/ess (battery) ==
  main_info_bus_in : Inport
  system_effort_in : Inport  Port=2
  system_flow_in : Inport  Port=3
  buscreator_system_bus_out1 : BusCreator  Inputs=2
  ctrl : Subsystem
      mask Display: disp('ess_ctrl_pngv_map_anl_PI_cstr.slx')
  memoryctrl : Memory
  plant : Subsystem
      mask Display: disp('ess_plant_pngv_map_anl_PI_cstr.slx')
  system_bus_out : Outport
  system_effort_out : Outport  Port=2
  system_flow_out : Outport  Port=3
  wires:
  [plant] -> buscreator_system_bus_out1/2  "plant"
  [ctrl] -> buscreator_system_bus_out1/1  "ctrl"
  buscreator_system_bus_out1/1 -> system_bus_out/1  "system_info_bus"
  system_flow_in/1 -> plant/4(in-flow-2)  "flow"
  system_effort_in/1 -> plant/3(in-effort-1)  "effort"
  plant/4(out-flow-13) -> system_flow_out/1  "flow"
  plant/3(out-effort-12) -> system_effort_out/1  "effort"
  plant/1(outport-system_info_bus) -> [plant]  "system_info_bus"
  memoryctrl/1 -> plant/2(aInport--2)  "ctrl_bus"
  plant/2(outport-plant_bus) -> ctrl/2(aInport--2)  "plant_bus"
  main_info_bus_in/1 -> plant/1(aInport--1), ctrl/1(inport-main_info_bus-1)  "main_info_bus"
  ctrl/2(outport-ctrl_bus) -> memoryctrl/1  "ctrl_bus"
  ctrl/1(outport-system_info_bus) -> [ctrl]  "system_info_bus"

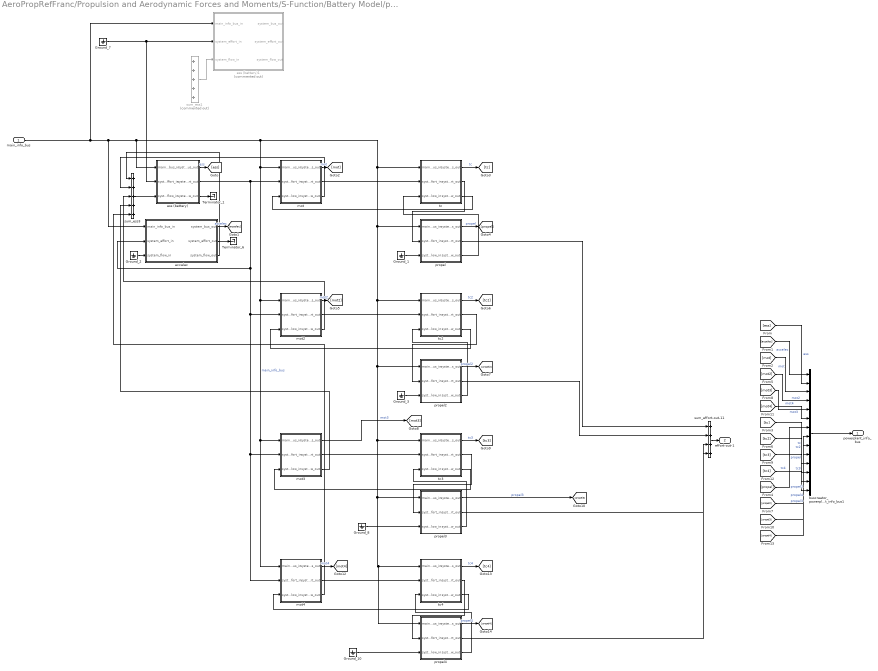
== system AeroPropRefFranc/Propulsion and Aerodynamic Forces and Moments/S-Function/Battery Model/powerplant ==
  main_info_bus : Inport
  Ground_{1..3,7..8,10} (6 alike) : Ground
  Terminator_1 : Terminator
  Terminator_6 : Terminator
  accelec : Subsystem
  buscreator_powerplant_info_bus1 : BusCreator  Inputs=14
  ess (battery) : Subsystem
  ess (battery)1 : Subsystem  Commented=on
  mot : Subsystem
  mot2 : Subsystem
  mot3 : Subsystem
  mot4 : Subsystem
  propel : Subsystem
  propel2 : Subsystem
  propel3 : Subsystem
  propel4 : Subsystem
  sum_effort-out-11 : Sum  Inputs=++++
  sum_ess1 : Sum  Commented=on  Inputs=+++++
  sum_ess3 : Sum  Inputs=+++++
  tc : Subsystem
  tc2 : Subsystem
  tc3 : Subsystem
  tc4 : Subsystem
  powerplant_info_bus : Outport  VectorParamsAs1DForOutWhenUnconnected=off
  effort-out-1 : Outport  Port=2  VectorParamsAs1DForOutWhenUnconnected=off
  wires:
  sum_ess1/1 -> ess (battery)1/3(system_flow_in)
  [tc4] -> buscreator_powerplant_info_bus1/14  "tc4"
  [tc3] -> buscreator_powerplant_info_bus1/13  "tc3"
  [tc2] -> buscreator_powerplant_info_bus1/12  "tc2"
  [tc] -> buscreator_powerplant_info_bus1/11  "tc"
  [propel4] -> buscreator_powerplant_info_bus1/10  "propel4"
  [propel3] -> buscreator_powerplant_info_bus1/9  "propel3"
  [propel2] -> buscreator_powerplant_info_bus1/8  "propel2"
  [propel] -> buscreator_powerplant_info_bus1/7  "propel"
  [mot4] -> buscreator_powerplant_info_bus1/6  "mot4"
  [mot3] -> buscreator_powerplant_info_bus1/5  "mot3"
  [mot2] -> buscreator_powerplant_info_bus1/4  "mot2"
  [mot] -> buscreator_powerplant_info_bus1/3  "mot"
  [ess] -> buscreator_powerplant_info_bus1/2  "ess"
  [accelec] -> buscreator_powerplant_info_bus1/1  "accelec"
  sum_effort-out-11/1 -> effort-out-1/1
  buscreator_powerplant_info_bus1/1 -> powerplant_info_bus/1
  tc4/1(system_bus_out) -> [tc4]  "tc4"
  tc3/1(system_bus_out) -> [tc3]  "tc3"
  tc2/1(system_bus_out) -> [tc2]  "tc2"
  tc/1(system_bus_out) -> [tc]  "tc"
  tc4/2(system_effort_out) -> propel4/2(system_effort_in)
  propel4/3(system_flow_out) -> tc4/3(system_flow_in)
  propel4/2(system_effort_out) -> sum_effort-out-11/4
  propel4/1(system_bus_out) -> [propel4]  "propel4"
  Ground_10/1 -> propel4/3(system_flow_in)
  tc3/2(system_effort_out) -> propel3/2(system_effort_in)
  propel3/3(system_flow_out) -> tc3/3(system_flow_in)
  propel3/2(system_effort_out) -> sum_effort-out-11/3
  propel3/1(system_bus_out) -> [propel3]  "propel3"
  Ground_8/1 -> propel3/3(system_flow_in)
  tc2/2(system_effort_out) -> propel2/2(system_effort_in)
  propel2/3(system_flow_out) -> tc2/3(system_flow_in)
  propel2/2(system_effort_out) -> sum_effort-out-11/2
  propel2/1(system_bus_out) -> [propel2]  "propel2"
  Ground_3/1 -> propel2/3(system_flow_in)
  tc/2(system_effort_out) -> propel/2(system_effort_in)
  propel/3(system_flow_out) -> tc/3(system_flow_in)
  propel/2(system_effort_out) -> sum_effort-out-11/1
  propel/1(system_bus_out) -> [propel]  "propel"
  Ground_1/1 -> propel/3(system_flow_in)
  tc4/3(system_flow_out) -> mot4/3(system_flow_in)
  mot4/3(system_flow_out) -> sum_ess3/5
  mot4/2(system_effort_out) -> tc4/2(system_effort_in)
  mot4/1(system_bus_out) -> [mot4]  "mot4"
  tc3/3(system_flow_out) -> mot3/3(system_flow_in)
  mot3/3(system_flow_out) -> sum_ess3/4
  mot3/2(system_effort_out) -> tc3/2(system_effort_in)
  mot3/1(system_bus_out) -> [mot3]  "mot3"
  tc2/3(system_flow_out) -> mot2/3(system_flow_in)
  mot2/3(system_flow_out) -> sum_ess3/3
  mot2/2(system_effort_out) -> tc2/2(system_effort_in)
  mot2/1(system_bus_out) -> [mot2]  "mot2"
  tc/3(system_flow_out) -> mot/3(system_flow_in)
  mot/3(system_flow_out) -> sum_ess3/2
  mot/2(system_effort_out) -> tc/2(system_effort_in)
  mot/1(system_bus_out) -> [mot]  "mot"
  sum_ess3/1 -> ess (battery)/3(system_flow_in)
  ess (battery)/3(system_flow_out) -> Terminator_1/1
  ess (battery)/1(system_bus_out) -> [ess]  "ess"
  Ground_7/1 -> ess (battery)1/2(system_effort_in), ess (battery)/2(system_effort_in)
  main_info_bus/1 -> ess (battery)1/1(main_info_bus_in), accelec/1(main_info_bus_in), ess (battery)/1(main_info_bus_in), tc/1(main_info_bus_in), propel/1(main_info_bus_in), tc2/1(main_info_bus_in), propel2/1(main_info_bus_in), tc3/1(main_info_bus_in), propel3/1(main_info_bus_in), tc4/1(main_info_bus_in), propel4/1(main_info_bus_in), mot/1(main_info_bus_in), mot2/1(main_info_bus_in), mot4/1(main_info_bus_in), mot3/1(main_info_bus_in)  "main_info_bus"
  ess (battery)/2(system_effort_out) -> mot/2(system_effort_in), accelec/2(system_effort_in), mot2/2(system_effort_in), mot4/2(system_effort_in), mot3/2(system_effort_in)
  accelec/3(system_flow_out) -> sum_ess3/1
  accelec/2(system_effort_out) -> Terminator_6/1
  accelec/1(system_bus_out) -> [accelec]  "accelec"
  Ground_2/1 -> accelec/3(system_flow_in)

== system AeroPropRefFranc/Propulsion and Aerodynamic Forces and Moments/S-Function/Engine Forces//Moments/RenameEngineForceMomentBus ==
  Bus Creator2 : BusCreator  Inputs=11  OutDataTypeStr=Bus: EngineFMBus
  Constant{1..4} (4 alike) : Constant  Value=zeros(3,1)
  Constant{5..11} (7 alike) : Constant  Value=zeros(1,SimIn.numEngines)
  Propulsion : Outport
  wires:
  Constant3/1 -> Bus Creator2/2  "Moment_b"
  Constant2/1 -> Bus Creator2/1  "Force_b"
  Bus Creator2/1 -> Propulsion/1  "Propulsion"
  Constant1/1 -> Bus Creator2/3  "H_b"
  Constant4/1 -> Bus Creator2/4  "Hdot_b"
  Constant7/1 -> Bus Creator2/7  "Mmotor_r"
  Constant8/1 -> Bus Creator2/8  "Hdot_r"
  Constant9/1 -> Bus Creator2/9  "H_r"
  Constant10/1 -> Bus Creator2/10  "Omega_r"
  Constant11/1 -> Bus Creator2/11  "AdvanceRatio"
  Constant5/1 -> Bus Creator2/5  "Fprop_r"
  Constant6/1 -> Bus Creator2/6  "Mprop_r"

== system AeroPropRefFranc/Propulsion and Aerodynamic Forces and Moments/S-Function/Propulsion Forces and Moments/Total Angular Momentum ==
  EngSpeed : Inport
  EngAccel : Inport  Port=2
  MATLAB Function : MATLAB Function  TreatAsAtomicUnit=on
  H_b : Outport
  Hdot_b : Outport  Port=2
  wires:
  MATLAB Function/2(Hdot_b) -> Hdot_b/1
  MATLAB Function/1(H_b) -> H_b/1
  EngAccel/1 -> MATLAB Function/2(EngAccel)
  EngSpeed/1 -> MATLAB Function/1(EngSpeed)

== system AeroPropRefFranc/Propulsion and Aerodynamic Forces and Moments/S-Function/Total Forces//Moments/RenameTotalForceMomentBus ==
  Bus Creator2 : BusCreator  Inputs=4  OutDataTypeStr=Bus: TotalFMBus
  Constant{2..5} (4 alike) : Constant  Value=zeros(3,1)
  Total : Outport
  wires:
  Bus Creator2/1 -> Total/1  "Total"
  Constant2/1 -> Bus Creator2/1  "Force_b"
  Constant3/1 -> Bus Creator2/2  "Moment_b"
  Constant4/1 -> Bus Creator2/3  "H_b"
  Constant5/1 -> Bus Creator2/4  "Hdot_b"

== system AeroPropRefFranc/Propulsion and Aerodynamic Forces and Moments/S-Function/Battery Model/accelec/plant ==
  aInport--1 : Inport
  aInport--2 : Inport  Port=2
  in-effort-2 : Inport  Port=3
  in-flow-3 : Inport  Port=4
  Ground_1 : Ground
  Ground_2 : Ground
  Terminator_1 : Terminator
  Terminator_2 : Terminator
  accelec_plant_const_pwrloss_volt_in_nokey : Subsystem
  parameter_out : Subsystem
  parameter_selection : Subsystem
  outport-system_info_bus : Outport
  aOutport--2 : Outport  Port=2
  out-effort-6 : Outport  Port=3
  out-flow-7 : Outport  Port=4
  wires:
  Ground_2/1 -> aOutport--2/1
  Ground_1/1 -> accelec_plant_const_pwrloss_volt_in_nokey/1(drv_key_on_dmd_simu)
  aInport--2/1 -> Terminator_2/1
  aInport--1/1 -> Terminator_1/1
  accelec_plant_const_pwrloss_volt_in_nokey/7(accelec_curr_in) -> out-flow-7/1
  accelec_plant_const_pwrloss_volt_in_nokey/6(accelec_volt_out) -> out-effort-6/1
  in-flow-3/1 -> accelec_plant_const_pwrloss_volt_in_nokey/3(accelec_curr_out)
  in-effort-2/1 -> accelec_plant_const_pwrloss_volt_in_nokey/2(accelec_volt_in)
  accelec_plant_const_pwrloss_volt_in_nokey/5(accelec_plant_curr_out_simu) -> parameter_out/5(inport-accelec_plant_curr_out_simu)
  accelec_plant_const_pwrloss_volt_in_nokey/4(accelec_plant_volt_out_simu) -> parameter_out/4(inport-accelec_plant_volt_out_simu)
  accelec_plant_const_pwrloss_volt_in_nokey/3(accelec_plant_curr_in_simu) -> parameter_out/3(inport-accelec_plant_curr_in_simu)
  accelec_plant_const_pwrloss_volt_in_nokey/2(accelec_plant_pwr_simu) -> parameter_out/2(inport-accelec_plant_pwr_simu)
  accelec_plant_const_pwrloss_volt_in_nokey/1(accelec_plant_volt_in_simu) -> parameter_out/1(inport-accelec_plant_volt_in_simu)
  parameter_out/1(outport-system_info_bus) -> outport-system_info_bus/1

== system AeroPropRefFranc/Propulsion and Aerodynamic Forces and Moments/S-Function/Battery Model/ess (battery)/ctrl ==
  inport-main_info_bus-1 : Inport
  aInport--2 : Inport  Port=2
  Terminator_1 : Terminator
  ess_ctrl_pngv_map_anl_PI_cstr : Subsystem
  parameter_out : Subsystem
  parameter_selection : Subsystem
  outport-system_info_bus : Outport
  outport-ctrl_bus : Outport  Port=2
  wires:
  aInport--2/1 -> Terminator_1/1
  parameter_selection/3(outport-ess_plant_soc_simu-3) -> ess_ctrl_pngv_map_anl_PI_cstr/3(ess_soc)
  parameter_selection/2(outport-ess_plant_curr_out_simu-2) -> ess_ctrl_pngv_map_anl_PI_cstr/2(ess_curr_out)
  parameter_selection/1(outport-ess_plant_volt_out_simu-1) -> ess_ctrl_pngv_map_anl_PI_cstr/1(ess_volt_out)
  ess_ctrl_pngv_map_anl_PI_cstr/4(ess_ctrl_curr_max_reg_simu) -> parameter_out/4(inport-ess_ctrl_curr_max_reg_simu)
  ess_ctrl_pngv_map_anl_PI_cstr/3(ess_ctrl_curr_max_pro_simu) -> parameter_out/3(inport-ess_ctrl_curr_max_pro_simu)
  ess_ctrl_pngv_map_anl_PI_cstr/2(ess_ctrl_pwr_max_reg_simu) -> parameter_out/2(inport-ess_ctrl_pwr_max_reg_simu)
  ess_ctrl_pngv_map_anl_PI_cstr/1(ess_ctrl_pwr_max_pro_simu) -> parameter_out/1(inport-ess_ctrl_pwr_max_pro_simu)
  parameter_out/2(outport-ctrl_bus) -> outport-ctrl_bus/1
  parameter_out/1(outport-system_info_bus) -> outport-system_info_bus/1
  inport-main_info_bus-1/1 -> parameter_selection/1(inport-main_info_bus-1)

== system AeroPropRefFranc/Propulsion and Aerodynamic Forces and Moments/S-Function/Battery Model/ess (battery)/plant ==
  aInport--1 : Inport
  aInport--2 : Inport  Port=2
  in-effort-1 : Inport  Port=3
  in-flow-2 : Inport  Port=4
  Terminator_1 : Terminator
  Terminator_2 : Terminator
  ess_plant_pngv_map_anl_PI_cstr : Subsystem
  parameter_out : Subsystem
  parameter_selection : Subsystem
  outport-system_info_bus : Outport
  outport-plant_bus : Outport  Port=2
  out-effort-12 : Outport  Port=3
  out-flow-13 : Outport  Port=4
  wires:
  aInport--2/1 -> Terminator_2/1
  aInport--1/1 -> Terminator_1/1
  ess_plant_pngv_map_anl_PI_cstr/13(ess_curr_in) -> out-flow-13/1
  ess_plant_pngv_map_anl_PI_cstr/12(ess_volt_out) -> out-effort-12/1
  in-flow-2/1 -> ess_plant_pngv_map_anl_PI_cstr/2(ess_curr_out)
  in-effort-1/1 -> ess_plant_pngv_map_anl_PI_cstr/1(ess_volt_in)
  ess_plant_pngv_map_anl_PI_cstr/9(ess_plant_curr_pol2_simu) -> parameter_out/9(inport-ess_plant_curr_pol2_simu)
  ess_plant_pngv_map_anl_PI_cstr/8(ess_plant_curr_pol1_simu) -> parameter_out/8(inport-ess_plant_curr_pol1_simu)
  ess_plant_pngv_map_anl_PI_cstr/7(ess_plant_rpol2_simu) -> parameter_out/7(inport-ess_plant_rpol2_simu)
  ess_plant_pngv_map_anl_PI_cstr/6(ess_plant_rpol1_simu) -> parameter_out/6(inport-ess_plant_rpol1_simu)
  ess_plant_pngv_map_anl_PI_cstr/5(ess_plant_rint_simu) -> parameter_out/5(inport-ess_plant_rint_simu)
  ess_plant_pngv_map_anl_PI_cstr/4(ess_plant_voc_simu) -> parameter_out/4(inport-ess_plant_voc_simu)
  ess_plant_pngv_map_anl_PI_cstr/3(ess_plant_volt_out_simu) -> parameter_out/3(inport-ess_plant_volt_out_simu)
  ess_plant_pngv_map_anl_PI_cstr/2(ess_plant_curr_out_simu) -> parameter_out/2(inport-ess_plant_curr_out_simu)
  ess_plant_pngv_map_anl_PI_cstr/11(ess_plant_impedance_simu) -> parameter_out/11(inport-ess_plant_impedance_simu)
  ess_plant_pngv_map_anl_PI_cstr/10(ess_plant_heat_out_simu) -> parameter_out/10(inport-ess_plant_heat_out_simu)
  ess_plant_pngv_map_anl_PI_cstr/1(ess_plant_soc_simu) -> parameter_out/1(inport-ess_plant_soc_simu)
  parameter_out/2(outport-plant_bus) -> outport-plant_bus/1
  parameter_out/1(outport-system_info_bus) -> outport-system_info_bus/1

== system AeroPropRefFranc/Propulsion and Aerodynamic Forces and Moments/S-Function/Battery Model/powerplant/accelec ==
  main_info_bus_in : Inport
  system_effort_in : Inport  Port=2
  system_flow_in : Inport  Port=3
  Ground_1 : Ground
  Terminator_1 : Terminator
  plant : Subsystem
      mask Display: disp('accelec_plant_const_pwrloss_volt_in_nokey.slx')
  system_bus_out : Outport
  system_effort_out : Outport  Port=2
  system_flow_out : Outport  Port=3
  wires:
  plant/2(aOutport--2) -> Terminator_1/1
  Ground_1/1 -> plant/2(aInport--2)
  [plant] -> system_bus_out/1  "plant"
  system_flow_in/1 -> plant/4(in-flow-3)
  system_effort_in/1 -> plant/3(in-effort-2)
  plant/4(out-flow-7) -> system_flow_out/1
  plant/3(out-effort-6) -> system_effort_out/1
  plant/1(outport-system_info_bus) -> [plant]
  main_info_bus_in/1 -> plant/1(aInport--1)

== system AeroPropRefFranc/Propulsion and Aerodynamic Forces and Moments/S-Function/Battery Model/powerplant/ess (battery) ==
  main_info_bus_in : Inport
  system_effort_in : Inport  Port=2
  system_flow_in : Inport  Port=3
  buscreator_system_bus_out1 : BusCreator  Inputs=2
  ctrl : Subsystem
      mask Display: disp('ess_ctrl_pngv_map_anl_PI_cstr.slx')
  memoryctrl : Memory
  plant : Subsystem
      mask Display: disp('ess_plant_pngv_map_anl_PI_cstr.slx')
  system_bus_out : Outport
  system_effort_out : Outport  Port=2
  system_flow_out : Outport  Port=3
  wires:
  [plant] -> buscreator_system_bus_out1/2  "plant"
  [ctrl] -> buscreator_system_bus_out1/1  "ctrl"
  buscreator_system_bus_out1/1 -> system_bus_out/1  "system_info_bus"
  system_flow_in/1 -> plant/4(in-flow-2)  "flow"
  system_effort_in/1 -> plant/3(in-effort-1)  "effort"
  plant/4(out-flow-13) -> system_flow_out/1  "flow"
  plant/3(out-effort-12) -> system_effort_out/1  "effort"
  plant/1(outport-system_info_bus) -> [plant]  "system_info_bus"
  memoryctrl/1 -> plant/2(aInport--2)  "ctrl_bus"
  plant/2(outport-plant_bus) -> ctrl/2(aInport--2)  "plant_bus"
  main_info_bus_in/1 -> plant/1(aInport--1), ctrl/1(inport-main_info_bus-1)  "main_info_bus"
  ctrl/2(outport-ctrl_bus) -> memoryctrl/1  "ctrl_bus"
  ctrl/1(outport-system_info_bus) -> [ctrl]  "system_info_bus"

== system AeroPropRefFranc/Propulsion and Aerodynamic Forces and Moments/S-Function/Battery Model/powerplant/ess (battery)1 ==
  main_info_bus_in : Inport
  system_effort_in : Inport  Port=2
  system_flow_in : Inport  Port=3
  buscreator_system_bus_out1 : BusCreator  Inputs=2
  ctrl : Subsystem
      mask Display: disp('ess_ctrl_pngv_map_anl_PI_cstr.slx')
  memoryctrl : Memory
  plant : Subsystem
      mask Display: disp('ess_plant_pngv_map_anl_PI_cstr.slx')
  system_bus_out : Outport
  system_effort_out : Outport  Port=2
  system_flow_out : Outport  Port=3
  wires:
  ctrl/1(outport-system_info_bus) -> [ctrl]  "system_info_bus"
  ctrl/2(outport-ctrl_bus) -> memoryctrl/1  "ctrl_bus"
  main_info_bus_in/1 -> ctrl/1(inport-main_info_bus-1), plant/1(aInport--1)  "main_info_bus"
  plant/2(outport-plant_bus) -> ctrl/2(aInport--2)  "plant_bus"
  memoryctrl/1 -> plant/2(aInport--2)  "ctrl_bus"
  plant/1(outport-system_info_bus) -> [plant]  "system_info_bus"
  plant/3(out-effort-12) -> system_effort_out/1  "effort"
  plant/4(out-flow-13) -> system_flow_out/1  "flow"
  system_effort_in/1 -> plant/3(in-effort-1)  "effort"
  system_flow_in/1 -> plant/4(in-flow-2)  "flow"
  buscreator_system_bus_out1/1 -> system_bus_out/1  "system_info_bus"
  [ctrl] -> buscreator_system_bus_out1/1  "ctrl"
  [plant] -> buscreator_system_bus_out1/2  "plant"

== system AeroPropRefFranc/Propulsion and Aerodynamic Forces and Moments/S-Function/Battery Model/powerplant/mot ==
  main_info_bus_in : Inport
  system_effort_in : Inport  Port=2
  system_flow_in : Inport  Port=3
  buscreator_system_bus_out1 : BusCreator  Inputs=2
  ctrl : Subsystem
  memoryctrl : Memory
  plant : Subsystem
      mask Display: disp('mot_plant_map_Pelec_funTW_volt_in.slx')
  system_bus_out : Outport
  system_effort_out : Outport  Port=2
  system_flow_out : Outport  Port=3
  wires:
  [plant] -> buscreator_system_bus_out1/2  "plant"
  [ctrl] -> buscreator_system_bus_out1/1  "ctrl"
  buscreator_system_bus_out1/1 -> system_bus_out/1  "system_info_bus"
  system_flow_in/1 -> plant/4(in-flow-3)  "flow"
  system_effort_in/1 -> plant/3(in-effort-2)  "effort"
  plant/4(out-flow-8) -> system_flow_out/1  "flow"
  plant/3(out-effort-7) -> system_effort_out/1  "effort"
  plant/1(outport-system_info_bus) -> [plant]  "system_info_bus"
  memoryctrl/1 -> plant/2(inport-ctrl_bus-2)  "ctrl_bus"
  plant/2(outport-plant_bus) -> ctrl/2(local_info_bus_in)  "plant_bus"
  main_info_bus_in/1 -> plant/1(aInport--1), ctrl/1(main_info_bus_in)  "main_info_bus"
  ctrl/2(local_info_bus_out) -> memoryctrl/1  "ctrl_bus"
  ctrl/1(system_bus_out) -> [ctrl]  "system_info_bus"
